simulink model "MICArraySimulation"  (R2020a)
settings: Solver=FixedStepAuto  StartTime=0.0  StopTime=Inf  FixedStep=2.2675736961451248E-5*1024  RelTol=1e-3
libraries: dspvision x2, dspsnks4 x1, dspsrcs4 x1
settings Model: Creator=albert  LastModifiedBy=albert

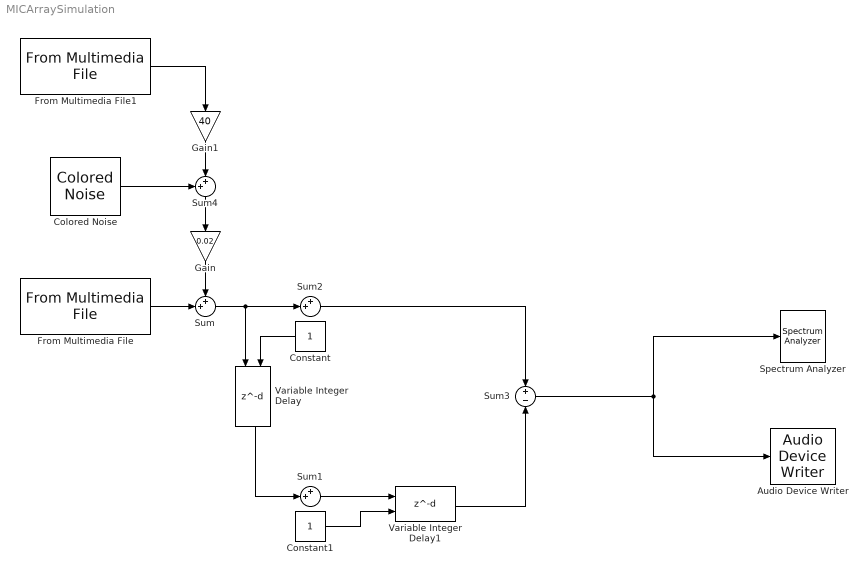
== system MICArraySimulation ==
  Audio Device Writer : dspsnks4/Audio Device Writer  Driver=DirectSound  Device=Default  InheritSampleRate=on  SampleRate=44100  BitDepth=16-bit integer  BufferSize=4096  NumBuffers=10  DefaultOutputChannelMapping=on  OutputChannelMapping=1:2  OutputNumUnderrunSamples=off  DriverIdx=1  DeviceWarnFlag=''
  Colored Noise : dspsrcs4/Colored Noise  Color=pink  InverseFrequencyPower=1  BoundedOutput=on  NumChannels=2  OutputDataType=double  SamplesPerFrame=1024  SampleTime=1  RandomStream=mt19937ar with seed  Seed=67  SimulateUsing=Interpreted execution
      settings: SourceProductBaseCode=DS
  Constant : Constant
  Constant1 : Constant
  From Multimedia File : dspvision/From Multimedia File  inputFilename=D:\CloudMusic\李悦君 - 梦伴.flac  readRange=[1 Inf]  loop=on  numPlays=inf  outputStreams=Audio only  videoDataType=single  audioDataType=double  inheritSampleTime=on  userDefinedSampleTime=1/30  noAudioOutput=off  isIntensityVideo=off  fourcc=RGB  colorVideoFormat=Separate color signals  outputEOF=off  dataOrg=Column-major  audioFrameSize=1024  computeAudioFrameSize=off  outSamplingMode=Sample based
  From Multimedia File1 : dspvision/From Multimedia File  inputFilename=D:\CloudMusic\Ghost.wav  readRange=[1 Inf]  loop=on  numPlays=inf  outputStreams=Audio only  videoDataType=single  audioDataType=double  inheritSampleTime=on  userDefinedSampleTime=1/30  noAudioOutput=off  isIntensityVideo=off  fourcc=RGB  colorVideoFormat=Separate color signals  outputEOF=off  dataOrg=Column-major  audioFrameSize=1024  computeAudioFrameSize=off  outSamplingMode=Sample based
  Gain : Gain  Gain=0.02
  Gain1 : Gain  Gain=40
  Spectrum Analyzer : SpectrumAnalyzer
  Sum{,1..2,4} (4 alike) : Sum  Inputs=++|
  Sum3 : Sum  Inputs=+|-
  Variable Integer Delay : Delay  DelayLengthSource=Input port
      settings: InputPortMap=u0,p1
  Variable Integer Delay1 : Delay  DelayLengthSource=Input port
      settings: InputPortMap=u0,p1
  wires:
  From Multimedia File/1 -> Sum/2
  Sum3/1 -> Audio Device Writer/1, Spectrum Analyzer/1
  Sum1/1 -> Variable Integer Delay1/1
  Constant/1 -> Variable Integer Delay/2
  Variable Integer Delay1/1 -> Sum3/2
  Constant1/1 -> Variable Integer Delay1/2
  Sum/1 -> Sum2/2, Variable Integer Delay/1
  Variable Integer Delay/1 -> Sum1/2
  Sum2/1 -> Sum3/1
  From Multimedia File1/1 -> Gain1/1
  Colored Noise/1 -> Sum4/1
  Sum4/1 -> Gain/1
  Gain1/1 -> Sum4/2
  Gain/1 -> Sum/1
